simulink model "mcb_microchip_pmsm_foc_sensorless_dsPIC33EP256MC506"  (R2021b)
settings: Solver=FixedStepDiscrete  StartTime=0.0  StopTime=10  FixedStep=Ts  RelTol=1e-3  EnableMultiTasking=on
InitFcn:
  | mcb_microchip_pmsm_foc_sensorless_dsPIC33_data;
values from neighbouring files (symbols this model uses):
  dataType = fixdt(1,16,14)    [mcb_microchip_pmsm_foc_sensorless_dsPIC33_data.m]    (also in mcb_pmsm_foc_sensorless_dsPIC33_data.m)
  dataType2 = fixdt(1,16,12)    [mcb_microchip_pmsm_foc_sensorless_dsPIC33_data.m]    (also in mcb_pmsm_foc_sensorless_dsPIC33_data.m)
  PI_params = mcb.internal.SetControllerParameters(pmsm,inverter,PU_System,T_pwm,Ts,Ts_speed)    [mcb_microchip_pmsm_foc_sensorless_dsPIC33_data.m]    (also in mcb_pmsm_foc_sensorless_dsPIC33_data.m)
  PU_System = mcb_SetPUSystem(pmsm,inverter)    [mcb_microchip_pmsm_foc_sensorless_dsPIC33_data.m]    (also in mcb_pmsm_foc_sensorless_dsPIC33_data.m)
  PWM_frequency = 20e3    (= 20000)    [mcb_microchip_pmsm_foc_sensorless_dsPIC33_data.m]    (also in mcb_pmsm_foc_sensorless_dsPIC33_data.m)
  Speed_openLoop_PU = 0.1    [mcb_microchip_pmsm_foc_sensorless_dsPIC33_data.m]    (also in mcb_pmsm_foc_sensorless_dsPIC33_data.m)
  Ts = T_pwm    (= 5e-05)    [mcb_microchip_pmsm_foc_sensorless_dsPIC33_data.m]    (also in mcb_pmsm_foc_sensorless_dsPIC33_data.m)
  Ts_speed = 30*Ts    (= 0.0015)    [mcb_microchip_pmsm_foc_sensorless_dsPIC33_data.m]    (also in mcb_pmsm_foc_sensorless_dsPIC33_data.m)
undefined symbols (not defined in the file or in its folder): A4, C5, D8, F1, inverter, P20, P53, P97, Pin, pmsm, PWMmax
libraries: MCHP_Blockset x16, mcbcontrolslib x13, simulink x9, mcbpositiondecoderlib x2, mcbplantlib x1, autolibpmsmexterior x1
(part 2 of 3)

== system mcb_microchip_pmsm_foc_sensorless_dsPIC33EP256MC506/Current Control/PWM Driver ==
  PWM (abc) : Inport
  Dead time Compensation : Bias  Bias=round( (inverter.deadtime/Ts) *PWMmax )
  Demux : Demux  Outputs=3
  PWM High Speed : MCHP_Blockset/PWM IO/PWM High Speed  pop1=[1]  chk1="[1  1  1  0  0]"  chkHL1="[1  1  1  1  1  1  1  1 ; 1  1  1  1  1  1  1  1]"  maxP1={ 'Ts','5e-05','5e-05','0.001','0.001','0.001','0.001','0.001';'0.001','0.001','1e-06','0.001','0.001','0.001','0.001','0.001'}  InitP2={ 'Ts','5e-05','5e-05','0.001','0.001','0.001','0.001','0.001';'0.001','0.001','0.001','0.001','0.001','0.001','0.001','0.001'}  chkP2="[0  0  0  1  1  1  1  1 ; 1  0  0  1  1  1  1  1]"  InitDC={ '4','4','4','50','50','50','50','50';'0.001','0.001','0.001','50','50','50','50','50'}  chkDC="[1  1  1  1  1  1  1  1 ; 0  0  0  1  1  1  1  1]"  InitPh={ '0','0','0','0.001','0.001','0.001','0.001','0.001';'0','0','0','0.001','0.001','0.001','0.001','0.001'}  chkPh="[0  0  0  1  1  1  1  1 ; 0  0  0  1  1  1  1  1]"  edSEvTrigx={ '0','-1','-1','-1','-1','-1','-1','-1'}  chkSEvTrigx="[0  0  0  1  1  1  1  1]"  popFlt="[2  2  2  1  1  1  1  1]"  popFltPin="[20  20  20   4   4   4   4   4]"  popFltPinRp="[1  1  1  1  1  1  1]"  popFltActivH="[2  2  2  1  1  1  1  1]"  popFltForceH="[2  2  2  2  2  2  2  2]"  popFltForceL="[1  1  1  1  1  1  1  1]"  chkFltBlkOut="[0  0  0  0  0  0  0  0]"  popIndepFaultMode="[1  1  1  1  1  1  1  1]"  popCurEnabled="[1  1  1  1  1  1  1  1]"  popCurPin="[4  31   4   4   4   4   4   4]"  popCurActiveH="[1  1  1  1  1  1  1  1]"  popCurForceH="[2  1  2  1  1  1  1  1]"  popCurForceL="[2  1  2  1  1  1  1  1]"  ChkCurBlkOut="[1  0  0  0  0  0  0  0]"  ChkCurBlkOutTime="[1  0  1  0  0  0  0  0]"  popBLANKSEL="[1  1  1  1  1  1  1  1]"  popBPHHBPHL="[1  1  1  1  1  1  1  1]"  popBPLHBPLL="[1  1  1  1  1  1  1  1]"  popFLTLEBEN_CLLEBEN="[1  1  1  1  1  1  1  1]"  popPHR_PHF="[2  1  1  1  1  1  1  1]"  popPLR_PLF="[3  1  1  1  1  1  1  1]"  edLEB={ '100e-9','50e-9','150e-9','50e-9','50e-9','50e-9','50e-9','50e-9'}  popDT="[1  1  1  3  3  3  3  3]"  edDTRx={ '0','0','0','1e-05','1e-05','1e-05','1e-05','1e-05'}  edAltDTRx={ 'inverter.deadtime','inverter.deadtime','inverter.deadtime','1e-05','1e-05','1e-05','1e-05','1e-05'}  S_INPUT="[5  5  5]"  S_INPUT_Size="[1  1  1]"  S_OUTPUT=[]  S_OUTPUT_Size=[]  S_DWORK_Type=[]  S_DWORK_Size=[]  ADC_VARTRIG={PWM Primary Special Event Trigger;6}  evalin_ws=PWMmax = 3499;PWM1max = 3499;PWM2max = 3499;PWM3max = 3499;  SampleTime=-1  ORDERING=None  MCHP_PORT={PWM1 Fault}{FLT32}4:0:B4;{PWM2 Fault}{FLT32}4:0:B4;{PWM3 Fault}{FLT32}4:0:B4;{PWM1H}{PWM1H}4:4:B14;{PWM1L}{PWM1L}4:4:B15;{PWM2H}{PWM2H}4:4:B12;{PWM2L}{PWM2L}4:4:B13;{PWM3H}{PWM3H}4:4:B10;{PWM3L}{PWM3L}4:4:B11;  MCHP_MASTERLINK=mcb_pmsm_foc_sensorless_dsPIC33EP256MC506/Hardware Init/Microchip Master  MCHP_VERSION=v3.38  Parameter50=0
      settings: SourceProductName=MPLAB Device Blocks for Simulink
  Saturation low side turn on errate workaround + errata for Phase shift (times 2) : Saturate  UpperLimit=PWMmax  LowerLimit=round( (inverter.deadtime/Ts) *PWMmax )* 2
  int to uint : DataTypeConversion  OutDataTypeStr=uint16  ConvertRealWorld=Stored Integer (SI)
  wires:
  int to uint/1 -> Saturation low side turn on errate workaround + errata for Phase shift (times 2)/1
  Dead time Compensation/1 -> int to uint/1
  PWM (abc)/1 -> Dead time Compensation/1
  Saturation low side turn on errate workaround + errata for Phase shift (times 2)/1 -> Demux/1
  Demux/1 -> PWM High Speed/1
  Demux/2 -> PWM High Speed/2
  Demux/3 -> PWM High Speed/3

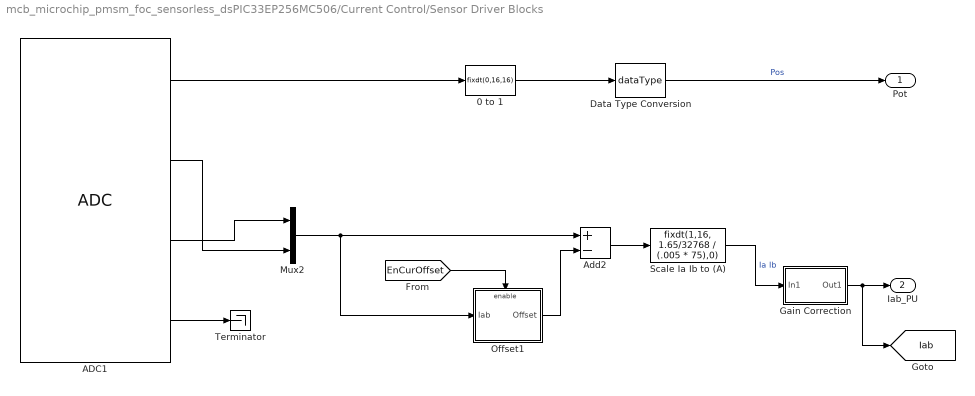
== system mcb_microchip_pmsm_foc_sensorless_dsPIC33EP256MC506/Current Control/Sensor Driver Blocks ==
  0 to 1 : DataTypeConversion  OutDataTypeStr=fixdt(0,16,16)  ConvertRealWorld=Stored Integer (SI)
  ADC1 : MCHP_Blockset/Analog IO/ADC  Priority=5  ADC_REF=1  Mode=10 bits (allows exact simultaneous sampling)  FORM=dddd dddd dddd 0000 ==> Unsigned fractional  ADC_R="< 5    kOhm"  nSAMPLECHANNELS=CH0 : CH1 : CH2 : CH3  nSAMPLECHANNELS_12bits=CH0 only  SIMULTANEOUS=Simultaneously on all Channels  ADxCSS=[13]  MUXA_CH0N=off  MUXA_CH123=Dynamic Options  MUXA_CH123_TXT=AN0 : AN1 : AN2  MUXB_CH0=AN13  MUXB_CH0N=on  MUXB_CH123=Dynamic Options  MUXB_CH123_TXT=AN0 : AN1 : AN2  SequenceRepeat=1  SequenceTiming=are done as fast as possible ; triggered by user define source  SSRC_SSRCG=Dynamic Options  SSRC_SSRCG_TXT=6  Update_BlockOutput=After each trig and conversion sequence  Trig_TimeStep=with each update of the ADC block output  ADC_DMA_CHANNEL=Use Interrupt instead of DMA  SampleTime=5e-05  Info=Total Time for Sample & Conversion : 4.4571e-06s including 3.4286e-07s (x 1) sample time.  MCHP_PORT={Analog Input 0}{AN0}15:2:A0;{Analog Input 1}{AN1}15:2:A1;{Analog Input 2}{AN2}15:2:B0;{Analog Input 13}{AN13}15:2:E13;  MCHP_MASTERLINK=mcb_pmsm_foc_sensorless_dsPIC33EP256MC506/Hardware Init/Microchip Master  ADC_TIMING=[4.4571428571428571832e-06]
      settings: SourceProductName=MPLAB Device Blocks for Simulink
  Add2 : Sum  Inputs=+-  OutDataTypeStr=int16  RndMeth=Zero
  Data Type Conversion : DataTypeConversion  OutDataTypeStr=dataType  RndMeth=Simplest
  Gain Correction : Subsystem
  Mux2 : Mux  Inputs=2
  Offset1 : Subsystem
  Scale Ia Ib to (A) : DataTypeConversion  OutDataTypeStr=fixdt(1,16, 1.65/32768 / (.005 * 75),0)  ConvertRealWorld=Stored Integer (SI)  RndMeth=Zero
  Terminator : Terminator
  Pot : Outport  VectorParamsAs1DForOutWhenUnconnected=off
  Iab_PU : Outport  Port=2  VectorParamsAs1DForOutWhenUnconnected=off
  tag scope: Iab=global
  wires:
  Mux2/1 -> Offset1/1(Iab), Add2/1
  0 to 1/1 -> Data Type Conversion/1
  [EnCurOffset] -> Offset1/Enable
  Data Type Conversion/1 -> Pot/1  "Pos"
  Add2/1 -> Scale Ia Ib to (A)/1
  ADC1/3 -> Mux2/1
  ADC1/1 -> 0 to 1/1
  Offset1/1(Offset) -> Add2/2
  ADC1/2 -> Mux2/2
  ADC1/4 -> Terminator/1
  Scale Ia Ib to (A)/1 -> Gain Correction/1(In1)  "Ia Ib"
  Gain Correction/1(Out1) -> [Iab], Iab_PU/1

== system mcb_microchip_pmsm_foc_sensorless_dsPIC33EP256MC506/Current Control/To Matlab Host  ==
  note: Note: Uncomment above blocks and comment Serial Send (below) to use Microchip's picgui interface to log hardware signals
  speed : Inport
  Data Store Read2 : DataStoreRead  DataStoreName=Speed_ref  IndexOptions=Index vector (dialog)  Indices=1  OutputSizes=1
  Gain : Gain  Gain=PU_System.N_base  OutDataTypeStr=uint16  RndMeth=Simplest
  Gain1 : Gain  Gain=PU_System.N_base  OutDataTypeStr=uint16
  Serial Send : Subsystem
  UART Tx-Matlab : MCHP_Blockset/BUS UART/UART Tx-Matlab  Commented=on  UART_REF=2  CHANNELS=[1 2]  AllOrNothing=off  SampleTime=.001  MCHP_MASTERLINK=mcb_pmsm_foc_sensorless_dsPIC33EP256MC506/Hardware Init/Microchip Master  MCHP_COMPILED_INFO="CompiledSampleTime= [0.0010000000000000000208   0 ];CompiledInportDataTypes=[  4   4 ];CompiledInportDataWidth=[1  1];"
      settings: SourceProductName=MPLAB Device Blocks for Simulink
  int to uint2 : DataTypeConversion  OutDataTypeStr=int16  ConvertRealWorld=Stored Integer (SI)
  int to uint3 : DataTypeConversion  OutDataTypeStr=int16  ConvertRealWorld=Stored Integer (SI)
  picgui Graphical interface : MCHP_Blockset/BUS UART/picgui Graphical interface  Commented=on  Nothing=0
      settings: SourceProductName=MPLAB Device Blocks for Simulink
  wires:
  speed/1 -> Serial Send/2(Speed_fb), Gain1/1
  Data Store Read2/1 -> Serial Send/1(Speed_ref), Gain/1
  Gain/1 -> int to uint3/1
  Gain1/1 -> int to uint2/1
  int to uint3/1 -> UART Tx-Matlab/1  "U2 CH1"
  int to uint2/1 -> UART Tx-Matlab/2  "U2 CH2"

== system mcb_microchip_pmsm_foc_sensorless_dsPIC33EP256MC506/Hardware Init/Open Board and Motor pages ==

== system mcb_microchip_pmsm_foc_sensorless_dsPIC33EP256MC506/Inverter and Motor/Codegeneration ==
  Duty_Cycles : Inport
  Ground : Ground
  Terminator : Terminator
  Feedbacks_Iab : Outport  VectorParamsAs1DForOutWhenUnconnected=off
  wires:
  Ground/1 -> Feedbacks_Iab/1
  Duty_Cycles/1 -> Terminator/1

== system mcb_microchip_pmsm_foc_sensorless_dsPIC33EP256MC506/Inverter and Motor/Simulation ==
  Duty_Cycles : Inport
  Inverter : Subsystem
  Load_Profile (Torque) : Subsystem
  Sensor_Measurements : Subsystem
  Surface Mount PMSM : autolibpmsmexterior/Surface Mount PMSM  port_config=Torque  sim_type=Discrete  Ts=Ts  P=pmsm.p  Rs=pmsm.Rs + inverter.R_board  Ldq_=pmsm.Ld  KConstText=Permanent flux linkage constant (lambda_pm):  lambda_pm=pmsm.FluxPM  Ke=159.9771  Kt=1.323  mechanical=[pmsm.J, pmsm.B, 0]  idq0=[0 0]  theta_init=0  omega_init=0  KConst=pmsm.FluxPM  lambda_pm_calc=pmsm.FluxPM  RefBlkName='autolibpmsmexterior/Surface Mount PMSM'  aMode=5  Ldq="[0.0002      0.0002]"
      settings: SourceProductBaseCode=PW,DR,MT,UV,VE
  Terminator : Terminator
  Terminator1 : Terminator
  Feedbacks_Iab : Outport  VectorParamsAs1DForOutWhenUnconnected=off
  wires:
  Surface Mount PMSM/3 -> Terminator/1
  Duty_Cycles/1 -> Inverter/1(Duty_abc)
  Surface Mount PMSM/2 -> Sensor_Measurements/1(PhaseCurr)  "Iabc"
  Sensor_Measurements/1(Iab_fb) -> Feedbacks_Iab/1
  Load_Profile (Torque)/1(Load_Trq) -> Surface Mount PMSM/1
  Inverter/1(Vabc) -> Surface Mount PMSM/2
  Surface Mount PMSM/1 -> Terminator1/1

== system mcb_microchip_pmsm_foc_sensorless_dsPIC33EP256MC506/Speed Control/PI_Controller_Speed ==
  N_ref : Inport
  N_fb : Inport  Port=2
  Enable : EnablePort
  AND : Logic  IconShape=distinctive  AllPortsSameDT=off  OutDataTypeStr=boolean
  Data Store Read : DataStoreRead  DataStoreName=Enable  IndexOptions=Index vector (dialog)  Indices=1  OutputSizes=1
  Data Store Read1 : DataStoreRead  DataStoreName=EnableFOC  IndexOptions=Index vector (dialog)  Indices=1  OutputSizes=1
  Discrete PI Controller with anti-windup & reset : mcbcontrolslib/Discrete PI Controller  with anti-windup & reset  UpperSaturationLimit=1  LowerSaturationLimit=-1
      settings: SourceProductBaseCode=MT
  Ki1 : Constant  Value=Ts_speed * PI_params.Ki_speed  OutDataTypeStr=dataType  SampleTime=-1
  Ki2 : Constant  Value=0  OutDataTypeStr=dataType  SampleTime=-1
  Kp1 : Constant  Value=PI_params.Kp_speed  OutDataTypeStr=dataType2  SampleTime=-1
  Logical Operator : Logic  Operator=NOT  IconShape=distinctive  AllPortsSameDT=off  OutDataTypeStr=boolean
  Sum : Sum  Inputs=|+-  OutDataTypeStr=Inherit: Same as first input
  Iq_ref : Outport  OutputWhenDisabled=reset  InitialOutput=0  VectorParamsAs1DForOutWhenUnconnected=off
  wires:
  Discrete PI Controller with anti-windup & reset/1 -> Iq_ref/1
  Ki1/1 -> Discrete PI Controller with anti-windup & reset/3
  Kp1/1 -> Discrete PI Controller with anti-windup & reset/2
  N_fb/1 -> Sum/2
  Sum/1 -> Discrete PI Controller with anti-windup & reset/1
  Logical Operator/1 -> Discrete PI Controller with anti-windup & reset/4
  Ki2/1 -> Discrete PI Controller with anti-windup & reset/5
  N_ref/1 -> Sum/1  "Speed_Ref"
  Data Store Read1/1 -> AND/1
  Data Store Read/1 -> AND/2
  AND/1 -> Logical Operator/1

== system mcb_microchip_pmsm_foc_sensorless_dsPIC33EP256MC506/Speed Control/Speed_Ref_Selector ==
  Speed_Ref : Inport
  Constant : Constant  Value=Speed_openLoop_PU  OutDataTypeStr=dataType
  Data Store Read1 : DataStoreRead  DataStoreName=EnClosedLoop  IndexOptions=Index vector (dialog)  Indices=1  OutputSizes=1
  Switch : Switch  Criteria=u2 > Threshold
  Zero_Cancellation : mcbcontrolslib/IIR Filter  VariantControl=Low Pass Filter  VariantSelect=Low-pass  Filter_constant=0.2  advancedSettings=off  Ts=50e-6  cutOff_freq=795.7747
      settings: SourceProductBaseCode=MT
  Speed_ref : Outport
  wires:
  Constant/1 -> Switch/3
  Data Store Read1/1 -> Switch/2
  Switch/1 -> Zero_Cancellation/1
  Speed_Ref/1 -> Switch/1
  Zero_Cancellation/1 -> Speed_ref/1

== system mcb_microchip_pmsm_foc_sensorless_dsPIC33EP256MC506/System Inputs/Adjust Pot output ==
  note: Toggle between enable and disable on press on Button S2
  In1 : Inport
  Add : Sum
  Button S2 : MCHP_Blockset/Digital IO/Digital Input  PORT=Dynamic Options  PORT_TXT="G   [ 6 : 9 ]"  PIN=7  PACK=off  SIMULTANEOUS=off  ORDERING=None  SampleTime=-1  MCHP_PORT={Digital In}{DIN}2:0:G7;  MCHP_MASTERLINK=mcb_pmsm_foc_sensorless_dsPIC33EP256MC506/Hardware Init/Microchip Master
      settings: SourceProductName=MPLAB Device Blocks for Simulink
  Constant : Constant  Value=0.3
  Gain : Gain  Gain=0.45
  Saturation : Saturate  UpperLimit=0.75  LowerLimit=0.3
  Triggered Subsystem : Subsystem  TreatAsAtomicUnit=on
  Out1 : Outport
  wires:
  In1/1 -> Gain/1
  Constant/1 -> Add/2
  Gain/1 -> Add/1
  Add/1 -> Saturation/1
  Saturation/1 -> Out1/1
  Button S2/1 -> Triggered Subsystem/Trigger

== system mcb_microchip_pmsm_foc_sensorless_dsPIC33EP256MC506/System Inputs/Sim ==
  Data Store Write : DataStoreWrite  DataStoreName=Enable  IndexOptions=Index vector (dialog)  Indices=1  OutputSizes=1
  Data Type Conversion : DataTypeConversion
  Enable : Step  Time=0.5  SampleTime=0
  Speed Ref (Sim) : Step  Time=4  Before=0.5  After=0.75  OutDataTypeStr=Inherit: Inherit via back propagation
  Out1 : Outport
  wires:
  Speed Ref (Sim)/1 -> Out1/1
  Data Type Conversion/1 -> Data Store Write/1
  Enable/1 -> Data Type Conversion/1

== system mcb_microchip_pmsm_foc_sensorless_dsPIC33EP256MC506/Current Control/Closed Loop Control/Clarke Transform ==
  a : Inport
  b : Inport  Port=2
  Data Type Duplicate : DataTypeDuplicate
  a16 : AlgorithmDescriptor  AlgorithmName=mcb_clarke  NumberOfInputs=2  InputBlockPath1=a  InputBlockPath2=b  InputBlockPath3=sine  InputBlockPath4=cos  ParameterBlockPath1=Constant  ParameterName1=Value  NumberOfOutputs=2  OutputBlockPath1=Alpha  OutputBlockPath2=Beta  AlgorithmParameterName1=AxisAlignment  AlgorithmParameterValue1=dAxis  AlgorithmParameterPrimary1=on
  a_plus_2b : Sum  Inputs=+++  RndMeth=Zero  OutDataTypeStr=Inherit: Same as first input
  one_by_sqrt3 : Gain  Gain=1/sqrt(3)  RndMeth=Zero  OutDataTypeStr=Inherit: Same as input
  Alpha : Outport  VectorParamsAs1DForOutWhenUnconnected=off
  Beta : Outport  Port=2  VectorParamsAs1DForOutWhenUnconnected=off
  wires:
  a/1 -> a_plus_2b/1, Alpha/1, Data Type Duplicate/1
  one_by_sqrt3/1 -> Beta/1
  a_plus_2b/1 -> one_by_sqrt3/1
  b/1 -> a_plus_2b/2, a_plus_2b/3, Data Type Duplicate/2

== system mcb_microchip_pmsm_foc_sensorless_dsPIC33EP256MC506/Current Control/Closed Loop Control/Current_Controllers ==
  Id : Inport
  Iq : Inport  Port=2
  Idq_ref_PU : Inport  Port=3
  DQ Limiter : mcbcontrolslib/DQ Limiter  Vmax=0.95
      settings: SourceProductBaseCode=MT
  Demux : Demux  Outputs=2
  Mux : Mux
  PI_Controller_Id : Subsystem
  PI_Controller_Iq : Subsystem
  Terminator : Terminator
  Vd_ref : Outport  VectorParamsAs1DForOutWhenUnconnected=off
  Vq_ref : Outport  Port=2  VectorParamsAs1DForOutWhenUnconnected=off
  Idq : Outport  Port=3  VectorParamsAs1DForOutWhenUnconnected=off
  wires:
  Iq/1 -> Mux/4, PI_Controller_Iq/2(I_fb)  "Iq_fb"
  Id/1 -> Mux/2, PI_Controller_Id/2(I_fb)  "Id_fb"
  Demux/1 -> Mux/1, PI_Controller_Id/1(I_ref)  "Id_Ref"
  Demux/2 -> Mux/3, PI_Controller_Iq/1(I_ref)  "Iq_Ref"
  Idq_ref_PU/1 -> Demux/1
  DQ Limiter/3 -> Terminator/1
  Mux/1 -> Idq/1
  PI_Controller_Iq/1(V_ref) -> DQ Limiter/2
  PI_Controller_Id/1(V_ref) -> DQ Limiter/1
  DQ Limiter/1 -> Vd_ref/1
  DQ Limiter/2 -> Vq_ref/1

== system mcb_microchip_pmsm_foc_sensorless_dsPIC33EP256MC506/Current Control/Closed Loop Control/Open_Loop_Control ==
  Pos_PU : Inport
  Speed_fb : Inport  Port=2
  Constant : Constant  Value=Speed_openLoop_PU  OutDataTypeStr=dataType
  Gain : Gain  Gain=Ts*PU_System.N_base*pmsm.p/60  OutDataTypeStr=Inherit: Same as input  ParamDataTypeStr=Inherit: Same as input
  OpentoClosed : Subsystem
  Position Generator : mcbcontrolslib/Position Generator  AngleOutput=Per-unit  ThetaSource=External  ThetaInput=5e-4  DataType=double  ExternalReset=none  Offset=0
      settings: SourceProductBaseCode=MT
  Switch : Switch  Criteria=u2 ~= 0
  Pos_PU_Out : Outport
  wires:
  Position Generator/1 -> Switch/3  "Eps"
  Gain/1 -> Position Generator/1
  Switch/1 -> Pos_PU_Out/1
  Pos_PU/1 -> Switch/1
  Constant/1 -> Gain/1
  Speed_fb/1 -> OpentoClosed/1(Speed_fb)
  OpentoClosed/1(EnClosedLoop) -> Switch/2

== system mcb_microchip_pmsm_foc_sensorless_dsPIC33EP256MC506/Current Control/Input Scaling/DC component removal ==
  SigIN : Inport
  Data Type Conversion1 : DataTypeConversion  OutDataTypeStr=dataType  RndMeth=Zero
  High Pass Filter 1 : Subsystem  Tag=FilterWizardSubSystem
  SigOUT : Outport
  wires:
  SigIN/1 -> High Pass Filter 1/1(Input)
  High Pass Filter 1/1(Output) -> Data Type Conversion1/1
  Data Type Conversion1/1 -> SigOUT/1

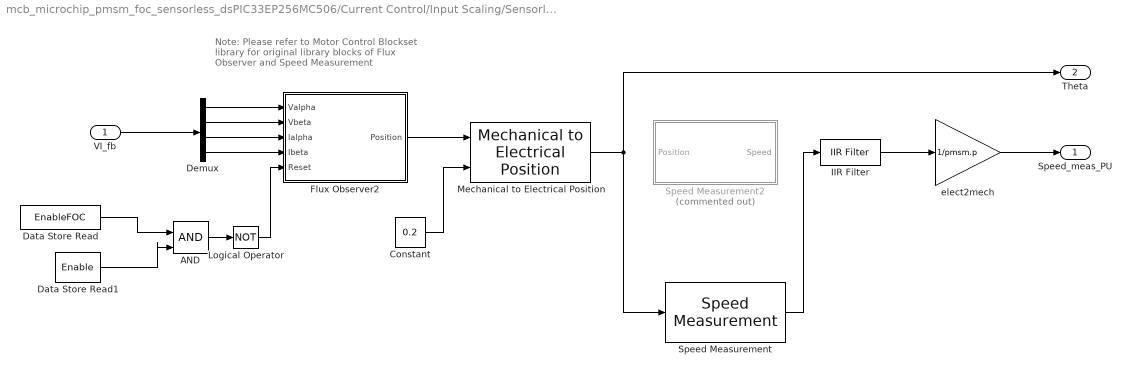
== system mcb_microchip_pmsm_foc_sensorless_dsPIC33EP256MC506/Current Control/Input Scaling/Sensorless ==
  note: Note: Please refer to Motor Control Blockset library for original library blocks of Flux Observer and Speed Measurement
  VI_fb : Inport
  AND : Logic  IconShape=distinctive  AllPortsSameDT=off  OutDataTypeStr=boolean
  Constant : Constant  Value=0.2  OutDataTypeStr=dataType
  Data Store Read : DataStoreRead  DataStoreName=EnableFOC  IndexOptions=Index vector (dialog)  Indices=1  OutputSizes=1
  Data Store Read1 : DataStoreRead  DataStoreName=Enable  IndexOptions=Index vector (dialog)  Indices=1  OutputSizes=1
  Demux : Demux
  Flux Observer2 : Subsystem  AncestorBlock=mcbpositiondecoderlib/Flux Observer  mask(Flux Observer){MotorSelection=PMSM, BlockInputUnit=Per-unit, PerUnitVoltage=PU_System.V_base, PerUnitCurrent=PU_System.I_base, PositionSelect=on, FluxSelect=off, TorqueSelect=off, PolePairs=4, StatorResistance=pmsm.Rs, StatorDAxisInductance=pmsm.Ld, StatorLeakageInductance=0.0068, RotorLeakageInductance=0.0068, MagnetizingInductance=0.0300, CutoffFreq=3.1863, BlockSampleTime=Ts, PositionUnit=Per-unit, PositionDatatype=dataType, FluxUnit=Weber, PerUnitFlux=0.1, FluxDatatype=single, TorqueUnit=Nm, PerUnitTorque=100, TorqueDatatype=single}
      mask prompts: MotorSelection "Motor selection:"; BlockInputUnit "Input units:"; PerUnitVoltage "Base voltage (V):"; PerUnitCurrent "Base current (A):"; PositionSelect "Position"; FluxSelect "Flux"; TorqueSelect "Torque"; PolePairs "Pole pairs:"; StatorResistance "Stator resistance (ohm):"; StatorDAxisInductance "Stator d-axis inductance (H):"; StatorLeakageInductance "Stator leakage inductance (H):"; RotorLeakageInductance "Rotor leakage inductance (H):"; MagnetizingInductance "Magnetizing inductance (H):"; CutoffFreq "Cutoff frequency (Hz):"; BlockSampleTime "Discrete step size (s):"; PositionUnit "Position unit:"; PositionDatatype "Position datatype:"; FluxUnit "Flux unit:"; PerUnitFlux "Per unit flux (Wb):"; FluxDatatype "Flux datatype:"; TorqueUnit "Torque unit:"; PerUnitTorque "Per unit torque (Nm):"; TorqueDatatype "Torque datatype:"
      mask help:
      | <p>Compute &#952;<sub>e</sub> (electrical position), &#936; (rotor magnetic flux), and T<sub>e</sub> (electromechanical torque) of a Permanent Magnet Synchronous Machine (PMSM) or Alternating Current Induction Machine (ACIM) from the voltages and currents in the stationary reference frame.
      | <br><br>
      | Use the Input units parameter to select the input unit of the block.
      | <br><br>
      | Use the Cutoff frequency parameter to set the lower cutoff frequency of the internal high Pass filter. Ensure that the values for Base voltage and Base current conform to the maximum applicable limits for the FO.</p>
      mask init:
      | mcb.internal.FOCb('MaskInitFcn', gcbh);
      mask Help: eval('mcb.internal.helpview(''fluxobserver'')')
      mask TypeOptions MotorSelection: PMSM | ACIM
      mask Callback MotorSelection: mcb.internal.FOCb('MotorSelectionMaskDisplay', gcbh);
      mask TypeOptions BlockInputUnit: SI unit | Per-unit
      mask Callback BlockInputUnit: mcb.internal.FOCb('MaskDisplay', gcbh);
      mask Callback PositionSelect: mcb.internal.FOCb('MaskDisplay', gcbh);
      mask Callback FluxSelect: mcb.internal.FOCb('MaskDisplay', gcbh);
      mask Callback TorqueSelect: mcb.internal.FOCb('MaskDisplay', gcbh);
      mask TypeOptions PositionUnit: Radians | Degrees | Per-unit
      mask TypeOptions FluxUnit: Weber | Per-unit
      mask Callback FluxUnit: mcb.internal.FOCb('MaskDisplay', gcbh);
      mask TypeOptions TorqueUnit: Nm | Per-unit
      mask Callback TorqueUnit: mcb.internal.FOCb('MaskDisplay', gcbh);
      mask DialogControl Container4 Prompt: Motor Parameters
      mask DialogControl Container7 Prompt: Block Output
      mask DialogControl Container8 Prompt: Datatypes
      mask Display:
      | color('black');
      | port_label('input',1, 'V_{\alpha}', 'interpreter', 'tex');
      | port_label('input',2, 'V_{\beta}', 'interpreter', 'tex');
      | port_label('input',3, 'I_{\alpha}', 'interpreter', 'tex');
      | port_label('input',4, 'I_{\beta}', 'interpreter', 'tex');
      | port_label('input',5, 'Rst', 'interpreter', 'tex');
      | port_label('output',1, '\theta_{e}', 'interpreter', 'tex');
      | %No Flux;
      | %No Torque;
      | fprintf('Flux\nObserver');
  IIR Filter : mcbcontrolslib/IIR Filter  VariantControl=Low Pass Filter  VariantSelect=Low-pass  Filter_constant=0.02  advancedSettings=off  Ts=50e-6  cutOff_freq=64.9612
      settings: SourceProductBaseCode=MT
  Logical Operator : Logic  Operator=NOT  IconShape=distinctive  AllPortsSameDT=off  OutDataTypeStr=boolean
  Mechanical to Electrical Position : mcbpositiondecoderlib/Mechanical to Electrical Position  NrPP=1  selectedRange=Per unit  MechOfstInputType=Input port  mechOffsetIn=0  maxAngleIn=1  InputDataType=dataType  VariantSelect=floating-point
      settings: SourceProductBaseCode=MT
  Speed Measurement : mcbpositiondecoderlib/Speed Measurement  PositionUnit=Per unit  PositionScalingDatatype=uint16  SpeedCalculationMode=Time interval for speed calculation  SampleTimeAsync=Ts  MaximumApplicationSpeed=1000  SpeedResolution=5e-6  DelayLength=20  MaximumMeasurableSpeed=-0.98352  MeasurableSpeedResolution=5.0304e-07  SpeedUnit=Per unit based on dialog  PerUnitSpeed=PU_System.N_base  SpeedDataType=dataType2
      settings: SourceProductBaseCode=MT
  Speed Measurement2 : Subsystem  Commented=on  AncestorBlock=mcbpositiondecoderlib/Speed Measurement  mask(Speed Measurement){PositionUnit=Per unit, SpeedCalculationMode=Time interval for speed calculation, SampleTimeAsync=Ts, MaximumApplicationSpeed=1000, SpeedResolution=5e-6, DelayLength=20, MaximumMeasurableSpeed=29999, MeasurableSpeedResolution=1.397e-05, SpeedUnit=Per unit based on dialog, PerUnitSpeed=PU_System.N_base, SpeedDataType=dataType2}
      mask prompts: PositionUnit "Position unit:"; SpeedCalculationMode "Speed calculation criteria:"; SampleTimeAsync "Discrete step size (s):"; MaximumApplicationSpeed "Maximum application speed (RPM):"; SpeedResolution "Speed resolution (RPM):"; DelayLength "Delays for speed calculation (number of samples):"; MaximumMeasurableSpeed "Maximum measurable speed (RPM):"; MeasurableSpeedResolution "Measurable speed resolution (RPM):"; SpeedUnit "Speed unit:"; PerUnitSpeed "Per unit speed (RPM):"; SpeedDataType "Speed data type:"
      mask help:
      | <p>Compute the speed from the rotor angular position.
      | <br>
      | <br>
      | &#952; (position) port accepts the position signal as either scalar fixed point or scalar floating point data type.</P>
      mask init:
      | mcb.internal.SpeedMeasurementCb('SpeedToCount', gcbh);
      | mcb.internal.SpeedMeasurementCb('SpeedUnit', gcbh);
      | mcb.internal.SpeedMeasurementCb('SetMaskDisplay', gcbh);
      mask Help: eval('mcb.internal.helpview(''speedmeasurement'')')
      mask TypeOptions PositionUnit: Radians | Degrees | Per unit
      mask Callback PositionUnit: mcb.internal.SpeedMeasurementCb('SpeedToCount', gcbh);
      mask TypeOptions SpeedCalculationMode: Maximum application speed | Speed resolution | Time interval for speed calculation
      mask Callback SpeedCalculationMode:
      | mcb.internal.SpeedMeasurementCb('SpeedCalculationModeCb', gcbh);
      | mcb.internal.SpeedMeasurementCb('MaskCalculation', gcbh,'SpeedCalculationMode');
      mask Callback SampleTimeAsync: mcb.internal.SpeedMeasurementCb('MaskCalculation', gcbh, 'SampleTimeAsync');
      mask Callback MaximumApplicationSpeed: mcb.internal.SpeedMeasurementCb('MaskCalculation', gcbh, 'MaximumApplicationSpeed');
      mask Callback SpeedResolution: mcb.internal.SpeedMeasurementCb('MaskCalculation', gcbh, 'SpeedResolution');
      mask Callback DelayLength: mcb.internal.SpeedMeasurementCb('MaskCalculation', gcbh, 'DelayLength');
      mask TypeOptions SpeedUnit: Degrees/Sec | Radians/Sec | RPM | Per unit based on maximum measurable speed | Per unit based on dialog
      mask Callback SpeedUnit: mcb.internal.SpeedMeasurementCb('PerUnitSpeedVisibility', gcbh);
      mask DialogControl General Prompt: Parameters
      mask Display:
      | color('black');
      | port_label('input',1, '\theta', 'texmode', 'on' );
      | port_label('output',1, '\omega', 'texmode', 'on' );
      | fprintf('Speed\nMeasurement');
  elect2mech : Gain  Gain=1/pmsm.p  OutDataTypeStr=dataType  RndMeth=Simplest
  Speed_meas_PU : Outport
  Theta : Outport  Port=2
  wires:
  Demux/3 -> Flux Observer2/3(Ialpha)
  Demux/1 -> Flux Observer2/1(Valpha)
  VI_fb/1 -> Demux/1
  Demux/4 -> Flux Observer2/4(Ibeta)
  Demux/2 -> Flux Observer2/2(Vbeta)
  IIR Filter/1 -> elect2mech/1
  elect2mech/1 -> Speed_meas_PU/1
  Speed Measurement/1 -> IIR Filter/1
  AND/1 -> Logical Operator/1
  Data Store Read/1 -> AND/1
  Data Store Read1/1 -> AND/2
  Flux Observer2/1(Position) -> Mechanical to Electrical Position/1
  Logical Operator/1 -> Flux Observer2/5(Reset)
  Mechanical to Electrical Position/1 -> Speed Measurement/1, Theta/1
  Constant/1 -> Mechanical to Electrical Position/2

== system mcb_microchip_pmsm_foc_sensorless_dsPIC33EP256MC506/Current Control/Output Scaling/Mode Selector ==
  Delay : Delay  DelayLength=1
  NOT : Logic  Operator=NOT  IconShape=distinctive  AllPortsSameDT=off  OutDataTypeStr=boolean
  Subsystem1 : Subsystem
  Up Counter : Subsystem
  CurrentOffsetEn : Outport
  wires:
  Up Counter/1(Count) -> Subsystem1/1(Count)
  Delay/1 -> NOT/1
  NOT/1 -> Up Counter/Enable
  Subsystem1/2(EnClosedLoop) -> Delay/1
  Subsystem1/1(Current Offset) -> CurrentOffsetEn/1

== system mcb_microchip_pmsm_foc_sensorless_dsPIC33EP256MC506/Current Control/Sensor Driver Blocks/Gain Correction ==
  In1 : Inport
  Demux : Demux  Outputs=2
  Gain : Gain  Gain=0.9615  RndMeth=Zero  OutDataTypeStr=Inherit: Same as input
  Mux : Mux  Inputs=2
  To Per-Unit : Gain  Gain=inverter.invertingAmp/PU_System.I_base  OutMin=-1  OutMax=1  OutDataTypeStr=fixdt(1,16)  RndMeth=Zero
  Out1 : Outport
  wires:
  Demux/1 -> Gain/1
  Demux/2 -> Mux/2
  To Per-Unit/1 -> Demux/1
  Gain/1 -> Mux/1
  Mux/1 -> Out1/1
  In1/1 -> To Per-Unit/1

== system mcb_microchip_pmsm_foc_sensorless_dsPIC33EP256MC506/Current Control/Sensor Driver Blocks/Offset1 ==
  Iab : Inport
  Enable : EnablePort
  Offset : Outport
  wires:
  Iab/1 -> Offset/1

== system mcb_microchip_pmsm_foc_sensorless_dsPIC33EP256MC506/Current Control/To Matlab Host /Serial Send ==
  Speed_ref : Inport
  Speed_fb : Inport  Port=2
  Debug_Data : Subsystem
  SCI_Tx : Subsystem
  wires:
  Debug_Data/1(Data_log) -> SCI_Tx/1(Data_Log)
  Speed_fb/1 -> Debug_Data/2(In2)
  Speed_ref/1 -> Debug_Data/1(In1)

== system mcb_microchip_pmsm_foc_sensorless_dsPIC33EP256MC506/Inverter and Motor/Simulation/Inverter ==
  Duty_abc : Inport
  Average-Value Inverter : mcbplantlib/Average-Value Inverter
  Constant2 : Constant  Value=inverter.V_dc  OutDataTypeStr=single  SampleTime=-1
  Data Type Conversion1 : DataTypeConversion  OutDataTypeStr=single  RndMeth=Simplest
  Vabc : Outport  VectorParamsAs1DForOutWhenUnconnected=off
  wires:
  Average-Value Inverter/1 -> Vabc/1
  Data Type Conversion1/1 -> Average-Value Inverter/1
  Duty_abc/1 -> Data Type Conversion1/1
  Constant2/1 -> Average-Value Inverter/2

== system mcb_microchip_pmsm_foc_sensorless_dsPIC33EP256MC506/Inverter and Motor/Simulation/Load_Profile (Torque) ==
  Constant : Constant  Value=0.2 * pmsm.T_rated  OutDataTypeStr=Inherit: Inherit via back propagation
  Data Type Conversion : DataTypeConversion  OutDataTypeStr=single
  IIR Filter : mcbcontrolslib/IIR Filter  VariantControl=Low Pass Filter  VariantSelect=Low-pass  Filter_constant=0.0001  advancedSettings=off  Ts=50e-6  cutOff_freq=0.31834
      settings: SourceProductBaseCode=MT
  Load_Trq : Outport  VectorParamsAs1DForOutWhenUnconnected=off
  wires:
  IIR Filter/1 -> Load_Trq/1
  Data Type Conversion/1 -> IIR Filter/1
  Constant/1 -> Data Type Conversion/1

== system mcb_microchip_pmsm_foc_sensorless_dsPIC33EP256MC506/Inverter and Motor/Simulation/Sensor_Measurements ==
  note: Delays
  note: Scaling
  PhaseCurr : Inport
  Data Type Conversion4 : DataTypeConversion  OutDataTypeStr=single  RndMeth=Simplest
  Delay1 : Delay  DelayLength=PI_params.delay_Currents
  Inverting OpAmp : Gain  Gain=1/PU_System.I_base  OutDataTypeStr=dataType  RndMeth=Simplest
  Selector : Selector  InputPortWidth=3  IndexOptions=Index vector (dialog)  Indices=[1 2]  OutputSizes=1
  Iab_fb : Outport  VectorParamsAs1DForOutWhenUnconnected=off
  wires:
  Selector/1 -> Inverting OpAmp/1
  PhaseCurr/1 -> Data Type Conversion4/1
  Data Type Conversion4/1 -> Delay1/1
  Delay1/1 -> Selector/1  "Iab_fb"
  Inverting OpAmp/1 -> Iab_fb/1

== system mcb_microchip_pmsm_foc_sensorless_dsPIC33EP256MC506/System Inputs/Adjust Pot output/Triggered Subsystem ==
  Trigger : TriggerPort  TriggerType=falling  VariantControl=Variant
  Data Store Write : DataStoreWrite  DataStoreName=Enable  IndexOptions=Index vector (dialog)  Indices=1  OutputSizes=1
  Delay : Delay  DelayLength=1  InitialCondition=0
  NOT : Logic  Operator=NOT  IconShape=distinctive  AllPortsSameDT=off  OutDataTypeStr=boolean
  wires:
  NOT/1 -> Data Store Write/1, Delay/1
  Delay/1 -> NOT/1

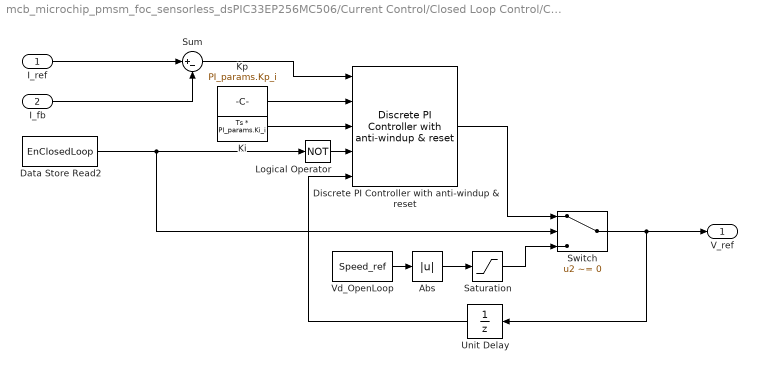
== system mcb_microchip_pmsm_foc_sensorless_dsPIC33EP256MC506/Current Control/Closed Loop Control/Current_Controllers/PI_Controller_Id ==
  I_ref : Inport
  I_fb : Inport  Port=2
  Abs : Abs  RndMeth=Simplest
  Data Store Read2 : DataStoreRead  DataStoreName=EnClosedLoop  IndexOptions=Index vector (dialog)  Indices=1  OutputSizes=1
  Discrete PI Controller with anti-windup & reset : mcbcontrolslib/Discrete PI Controller  with anti-windup & reset  UpperSaturationLimit=1  LowerSaturationLimit=-1
      settings: SourceProductBaseCode=MT
  Ki : Constant  Value=Ts * PI_params.Ki_i  OutDataTypeStr=dataType  SampleTime=-1
  Kp : Constant  Value=PI_params.Kp_i  OutDataTypeStr=dataType2  SampleTime=-1
  Logical Operator : Logic  Operator=NOT  IconShape=distinctive  AllPortsSameDT=off  OutDataTypeStr=boolean
  Saturation : Saturate  UpperLimit=0.15  LowerLimit=0.15  RndMeth=Simplest
  Sum : Sum  Inputs=|+-  OutDataTypeStr=Inherit: Same as first input
  Switch : Switch  Criteria=u2 ~= 0  RndMeth=Simplest
  Unit Delay : UnitDelay  SampleTime=-1  HasFrameUpgradeWarning=on
  Vd_OpenLoop : DataStoreRead  DataStoreName=Speed_ref  IndexOptions=Index vector (dialog)  Indices=1  OutputSizes=1
  V_ref : Outport  VectorParamsAs1DForOutWhenUnconnected=off
  wires:
  I_ref/1 -> Sum/1
  I_fb/1 -> Sum/2
  Data Store Read2/1 -> Switch/2, Logical Operator/1
  Sum/1 -> Discrete PI Controller with anti-windup & reset/1
  Kp/1 -> Discrete PI Controller with anti-windup & reset/2
  Ki/1 -> Discrete PI Controller with anti-windup & reset/3
  Logical Operator/1 -> Discrete PI Controller with anti-windup & reset/4
  Saturation/1 -> Switch/3
  Switch/1 -> Unit Delay/1, V_ref/1
  Discrete PI Controller with anti-windup & reset/1 -> Switch/1
  Unit Delay/1 -> Discrete PI Controller with anti-windup & reset/5
  Vd_OpenLoop/1 -> Abs/1
  Abs/1 -> Saturation/1

== system mcb_microchip_pmsm_foc_sensorless_dsPIC33EP256MC506/Current Control/Closed Loop Control/Current_Controllers/PI_Controller_Iq ==
  I_ref : Inport
  I_fb : Inport  Port=2
  Data Store Read1 : DataStoreRead  DataStoreName=EnClosedLoop  IndexOptions=Index vector (dialog)  Indices=1  OutputSizes=1
  Discrete PI Controller with anti-windup & reset : mcbcontrolslib/Discrete PI Controller  with anti-windup & reset  UpperSaturationLimit=1  LowerSaturationLimit=-1
      settings: SourceProductBaseCode=MT
  Ki : Constant  Value=Ts * PI_params.Ki_i  OutDataTypeStr=dataType  SampleTime=-1
  Kp : Constant  Value=PI_params.Kp_i  OutDataTypeStr=dataType2  SampleTime=-1
  Logical Operator : Logic  Operator=NOT  IconShape=distinctive  AllPortsSameDT=off  OutDataTypeStr=boolean
  Sum : Sum  Inputs=|+-  OutDataTypeStr=Inherit: Same as first input
  Switch : Switch  Criteria=u2 ~= 0  RndMeth=Simplest
  Unit Delay : UnitDelay  SampleTime=-1  HasFrameUpgradeWarning=on
  Vq_OpenLoop : Constant  Value=0  OutDataTypeStr=dataType  SampleTime=-1
  V_ref : Outport  VectorParamsAs1DForOutWhenUnconnected=off
  wires:
  I_fb/1 -> Sum/2
  I_ref/1 -> Sum/1
  Kp/1 -> Discrete PI Controller with anti-windup & reset/2
  Sum/1 -> Discrete PI Controller with anti-windup & reset/1
  Ki/1 -> Discrete PI Controller with anti-windup & reset/3
  Logical Operator/1 -> Discrete PI Controller with anti-windup & reset/4
  Data Store Read1/1 -> Switch/2, Logical Operator/1
  Vq_OpenLoop/1 -> Switch/3
  Discrete PI Controller with anti-windup & reset/1 -> Switch/1
  Unit Delay/1 -> Discrete PI Controller with anti-windup & reset/5
  Switch/1 -> Unit Delay/1, V_ref/1

== system mcb_microchip_pmsm_foc_sensorless_dsPIC33EP256MC506/Current Control/Closed Loop Control/Open_Loop_Control/OpentoClosed ==
  Speed_fb : Inport
  Chart : Stateflow chart  TreatAsAtomicUnit=on
  Data Store Read5 : DataStoreRead  DataStoreName=Enable  IndexOptions=Index vector (dialog)  Indices=1  OutputSizes=1
  Data Store Write1 : DataStoreWrite  DataStoreName=EnSpeedCtrl  IndexOptions=Index vector (dialog)  Indices=1  OutputSizes=1
  Data Store Write2 : DataStoreWrite  DataStoreName=EnClosedLoop  IndexOptions=Index vector (dialog)  Indices=1  OutputSizes=1
  Data Type Conversion : DataTypeConversion  OutDataTypeStr=boolean  RndMeth=Simplest
  Data Type Conversion1 : DataTypeConversion
  Enable Closed Loop : Constant  OutDataTypeStr=uint16
  Enable Closed Loop1 : Constant  Value=Speed_openLoop_PU*0.8  OutDataTypeStr=dataType
  Open Loop Start-up : Constant  Value=0  OutDataTypeStr=uint16
  Switch2 : Switch  Criteria=u2 > Threshold  Threshold=1
  EnClosedLoop : Outport
  wires:
  Open Loop Start-up/1 -> Switch2/3
  Data Store Read5/1 -> Chart/3(En)
  Chart/1(Mode) -> Switch2/2
  Switch2/1 -> Data Type Conversion/1
  Speed_fb/1 -> Chart/2(SpeedFb)
  Enable Closed Loop/1 -> Switch2/1
  Enable Closed Loop1/1 -> Chart/1(Limit)
  Data Type Conversion/1 -> EnClosedLoop/1, Data Store Write2/1
  Chart/2(SpeedCtrl) -> Data Type Conversion1/1
  Data Type Conversion1/1 -> Data Store Write1/1

== system mcb_microchip_pmsm_foc_sensorless_dsPIC33EP256MC506/Current Control/Input Scaling/DC component removal/High Pass Filter 1 ==
  Input : Inport
  A2Delay1 : Delay  DelayLength=1  InitialCondition=0
  B2Delay1 : Delay  DelayLength=1  InitialCondition=0
  CastStates1 : DataTypeConversion  OutDataTypeStr=fixdt(1,16,15)  SaturateOnIntegerOverflow=on  RndMeth=Zero
  ConvertIn : DataTypeConversion  OutDataTypeStr=fixdt(1,16,15)  RndMeth=Nearest  SaturateOnIntegerOverflow=on
  ConvertScale1 : DataTypeConversion  OutDataTypeStr=fixdt(1,16,15)  SaturateOnIntegerOverflow=on  RndMeth=Zero
  SumA21 : Sum  Inputs=|+-  AccumDataTypeStr=fixdt(1,32,27)  OutDataTypeStr=fixdt(1,32,27)  RndMeth=Zero  SaturateOnIntegerOverflow=on
  SumB21 : Sum  Inputs=|++  AccumDataTypeStr=fixdt(1,32,28)  OutDataTypeStr=fixdt(1,32,28)  RndMeth=Zero  SaturateOnIntegerOverflow=on
  a(2)(1) : Gain  Gain=-0.993965307066752457  ParamDataTypeStr=fixdt(1,16,14)  OutDataTypeStr=fixdt(1,32,29)  RndMeth=Zero  SaturateOnIntegerOverflow=on
  b(1)(1) : Gain  Gain=0.996982653533543983  ParamDataTypeStr=fixdt(1,16,15)  OutDataTypeStr=fixdt(1,32,30)  RndMeth=Zero  SaturateOnIntegerOverflow=on
  b(2)(1) : Gain  Gain=-0.996982653533543983  ParamDataTypeStr=fixdt(1,16,15)  OutDataTypeStr=fixdt(1,32,30)  RndMeth=Zero  SaturateOnIntegerOverflow=on
  s(2) : Gain  Gain=0.99999999999983169  ParamDataTypeStr=fixdt(1,16,15)  OutDataTypeStr=fixdt(1,16,11)  RndMeth=Zero  SaturateOnIntegerOverflow=on
  Output : Outport
  wires:
  Input/1 -> ConvertIn/1
  ConvertScale1/1 -> b(1)(1)/1, B2Delay1/1
  b(1)(1)/1 -> SumB21/1
  SumB21/1 -> SumA21/1
  SumA21/1 -> CastStates1/1
  CastStates1/1 -> s(2)/1, A2Delay1/1
  B2Delay1/1 -> b(2)(1)/1
  b(2)(1)/1 -> SumB21/2
  a(2)(1)/1 -> SumA21/2
  A2Delay1/1 -> a(2)(1)/1
  s(2)/1 -> Output/1
  ConvertIn/1 -> ConvertScale1/1

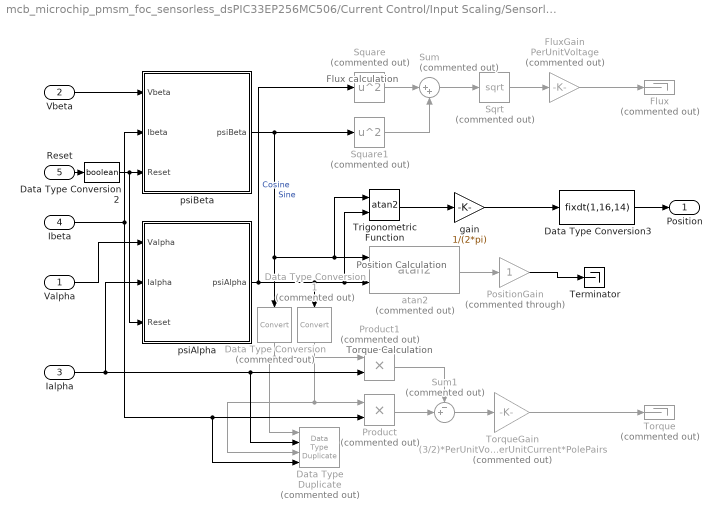
== system mcb_microchip_pmsm_foc_sensorless_dsPIC33EP256MC506/Current Control/Input Scaling/Sensorless/Flux Observer2 ==
  note: Flux calculation
  note: Position Calculation
  note: Torque Calculation
  Valpha : Inport  SampleTime=BlockSampleTime
  Vbeta : Inport  Port=2  SampleTime=BlockSampleTime
  Ialpha : Inport  Port=3  SampleTime=BlockSampleTime
  Ibeta : Inport  Port=4  SampleTime=BlockSampleTime
  Reset : Inport  Port=5  SampleTime=BlockSampleTime
  Data Type Duplicate : DataTypeDuplicate  Commented=on  NumInputPorts=4
  Data Type Conversion : DataTypeConversion  Commented=on  RndMeth=Simplest
  Data Type Conversion1 : DataTypeConversion  Commented=on  RndMeth=Simplest
  Data Type Conversion2 : DataTypeConversion  OutDataTypeStr=boolean  RndMeth=Simplest
  Data Type Conversion3 : DataTypeConversion  OutDataTypeStr=fixdt(1,16,14)  RndMeth=Simplest
  Flux : Terminator  Commented=on
  FluxGain : Gain  Commented=on  Gain=PerUnitVoltage  OutDataTypeStr=FluxDatatype  RndMeth=Simplest
  PositionGain : Gain  Commented=through  OutDataTypeStr=PositionDatatype  RndMeth=Simplest
  Product : Product  Commented=on  RndMeth=Simplest  OutDataTypeStr=Inherit: Same as first input
  Product1 : Product  Commented=on  RndMeth=Simplest  OutDataTypeStr=Inherit: Same as first input
  Sqrt : Sqrt  Commented=on  RndMeth=Simplest  IntermediateResultsDataTypeStr=Inherit: Inherit from input  SaturateOnIntegerOverflow=on
  Square : Math  Commented=on  Operator=square  RndMeth=Simplest  SaturateOnIntegerOverflow=on
  Square1 : Math  Commented=on  Operator=square  RndMeth=Simplest  SaturateOnIntegerOverflow=on
  Sum : Sum  Commented=on  Inputs=|++
  Sum1 : Sum  Commented=on  Inputs=-+|
  Terminator : Terminator
  Torque : Terminator  Commented=on
  TorqueGain : Gain  Commented=on  Gain=(3/2)*PerUnitVoltage*PerUnitCurrent*PolePairs  OutDataTypeStr=TorqueDatatype
  Trigonometric Function : Trigonometry  Operator=atan2  ApproximationMethod=CORDIC
  atan2 : mcbcontrolslib/atan2  Commented=on  outputUnit=PerUnit
      settings: SourceProductBaseCode=MT
  gain : Gain  Gain=1/(2*pi)  OutDataTypeStr=fixdt(0,16,16)  RndMeth=Simplest
  psiAlpha : Subsystem
  psiBeta : Subsystem
  Position : Outport
  wires:
  Data Type Conversion2/1 -> psiBeta/3(Reset), psiAlpha/3(Reset)
  Data Type Conversion1/1 -> Product/1, Data Type Duplicate/3
  Data Type Conversion/1 -> Product1/1, Data Type Duplicate/1
  atan2/1 -> PositionGain/1
  Sqrt/1 -> FluxGain/1
  Square1/1 -> Sum/2
  Sum/1 -> Sqrt/1
  Square/1 -> Sum/1
  FluxGain/1 -> Flux/1
  Sum1/1 -> TorqueGain/1
  Product1/1 -> Sum1/1
  Ialpha/1 -> Product1/2, Data Type Duplicate/2, psiAlpha/2(Ialpha)
  Product/1 -> Sum1/2
  TorqueGain/1 -> Torque/1
  Reset/1 -> Data Type Conversion2/1
  Vbeta/1 -> psiBeta/1(Vbeta)
  Ibeta/1 -> Product/2, Data Type Duplicate/4, psiBeta/2(Ibeta)
  Valpha/1 -> psiAlpha/1(Valpha)
  PositionGain/1 -> Terminator/1
  Trigonometric Function/1 -> gain/1
  gain/1 -> Data Type Conversion3/1
  Data Type Conversion3/1 -> Position/1
  psiBeta/1(psiBeta) -> Data Type Conversion/1, atan2/1, Trigonometric Function/1, Square1/1  "Sine"
  psiAlpha/1(psiAlpha) -> Square/1, Data Type Conversion1/1, Trigonometric Function/2, atan2/2  "Cosine"

== system mcb_microchip_pmsm_foc_sensorless_dsPIC33EP256MC506/Current Control/Input Scaling/Sensorless/Speed Measurement2 ==
  note: Speed measurement
  note: Speed measurement
  Position : Inport  SampleTime=SampleTimeAsync
  Data Type Conversion1 : DataTypeConversion  OutDataTypeStr=int32  ConvertRealWorld=Stored Integer (SI)
  Delay : Delay  Commented=on  DelayLength=DelayLength  UseCircularBuffer=on
  Delay1 : Delay  DelayLength=DelayLength  UseCircularBuffer=on
  Shift Arithmetic1 : ArithShift  BinPtShiftNumber=14  BitShiftDirection=Left
  Shift Arithmetic2 : ArithShift  BitShiftNumber=18  BitShiftDirection=Left
  SpeedCount : Sum  Commented=on  Inputs=+-|  OutDataTypeStr=int32  RndMeth=Simplest
  SpeedCount1 : Sum  Inputs=+-|  OutDataTypeStr=int32  RndMeth=Simplest
  SpeedGain : Gain  Commented=on  Gain=60/(DelayLength*SampleTimeAsync(1)*PU_System.N_base*4294967296)  ParamDataTypeStr=fixdt(0,16)  OutDataTypeStr=fixdt(1,16,12)  RndMeth=Simplest
  SpeedGain1 : Gain  Gain=60/(DelayLength*SampleTimeAsync(1)*PU_System.N_base*4294967296)  ParamDataTypeStr=fixdt(0,16)  OutDataTypeStr=fixdt(1,16,12)  RndMeth=Simplest
  SpeedToCount : Gain  Commented=on  Gain=uint32(4294967296/1)  ParamDataTypeStr=uint32  OutDataTypeStr=uint32  RndMeth=Simplest
  Speed : Outport  VectorParamsAs1DForOutWhenUnconnected=off
  wires:
  Data Type Conversion1/1 -> Shift Arithmetic2/1
  Shift Arithmetic1/1 -> Data Type Conversion1/1
  Position/1 -> SpeedToCount/1, Shift Arithmetic1/1
  Delay1/1 -> SpeedCount1/2
  Shift Arithmetic2/1 -> SpeedCount1/1, Delay1/1
  SpeedCount1/1 -> SpeedGain1/1
  SpeedCount/1 -> SpeedGain/1
  SpeedToCount/1 -> Delay/1, SpeedCount/1
  Delay/1 -> SpeedCount/2
  SpeedGain1/1 -> Speed/1

== system mcb_microchip_pmsm_foc_sensorless_dsPIC33EP256MC506/Current Control/Output Scaling/Mode Selector/Subsystem1 ==
  Count : Inport
  Compare To Constant : simulink/Logic and Bit Operations/Compare To Constant  relop=>=  const=1  OutDataTypeStr=boolean
  Compare To Constant1 : simulink/Logic and Bit Operations/Compare To Constant  relop=<  const=1  OutDataTypeStr=boolean
  Data Store Write1 : DataStoreWrite  DataStoreName=EnableFOC  IndexOptions=Index vector (dialog)  Indices=1  OutputSizes=1
  Gain : Gain  Gain=1/(2*PWM_frequency)  OutDataTypeStr=dataType2  RndMeth=Simplest
  Current Offset : Outport
  EnClosedLoop : Outport  Port=2
  tag scope: EnCurOffset=global
  wires:
  Count/1 -> Gain/1
  Gain/1 -> Compare To Constant1/1, Compare To Constant/1
  Compare To Constant/1 -> Data Store Write1/1, EnClosedLoop/1
  Compare To Constant1/1 -> [EnCurOffset], Current Offset/1

== system mcb_microchip_pmsm_foc_sensorless_dsPIC33EP256MC506/Current Control/Output Scaling/Mode Selector/Up Counter ==
  Enable : EnablePort  StatesWhenEnabling=reset
  Add1 : Sum  SaturateOnIntegerOverflow=on
  Constant : Constant  OutDataTypeStr=uint32
  Delay : Delay  DelayLength=1
  Count : Outport  InitialOutput=0
  wires:
  Delay/1 -> Add1/2
  Add1/1 -> Count/1, Delay/1
  Constant/1 -> Add1/1

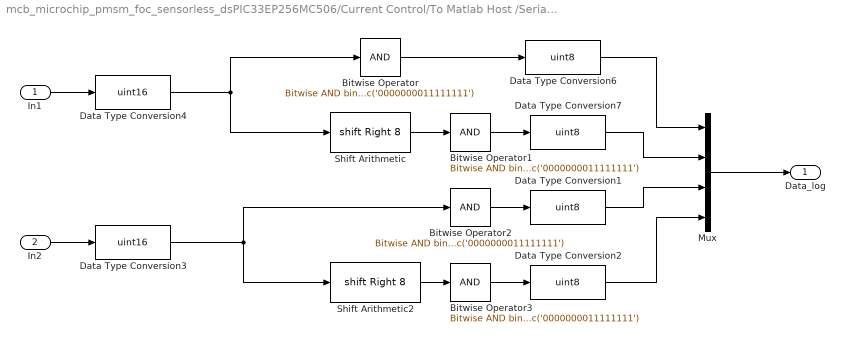
== system mcb_microchip_pmsm_foc_sensorless_dsPIC33EP256MC506/Current Control/To Matlab Host /Serial Send/Debug_Data ==
  In1 : Inport
  In2 : Inport  Port=2
  Bitwise Operator{,1..3} (4 alike) : simulink/Logic and Bit Operations/Bitwise Operator  logicop=AND  UseBitMask=on  BitMask=bin2dec('0000000011111111')  BitMaskRealWorld=Stored Integer
  Data Type Conversion{1..2,6..7} (4 alike) : DataTypeConversion  OutDataTypeStr=uint8  RndMeth=Simplest
  Data Type Conversion3 : DataTypeConversion  OutDataTypeStr=uint16  ConvertRealWorld=Stored Integer (SI)  RndMeth=Simplest
  Data Type Conversion4 : DataTypeConversion  OutDataTypeStr=uint16  ConvertRealWorld=Stored Integer (SI)  RndMeth=Simplest
  Mux : Mux
  Shift Arithmetic : ArithShift  BitShiftNumber=8  BitShiftDirection=Right
  Shift Arithmetic2 : ArithShift  BitShiftNumber=8  BitShiftDirection=Right
  Data_log : Outport
  wires:
  Data Type Conversion3/1 -> Bitwise Operator2/1, Shift Arithmetic2/1
  Bitwise Operator3/1 -> Data Type Conversion2/1
  Shift Arithmetic2/1 -> Bitwise Operator3/1
  Bitwise Operator1/1 -> Data Type Conversion7/1
  Data Type Conversion2/1 -> Mux/4
  Shift Arithmetic/1 -> Bitwise Operator1/1
  Bitwise Operator/1 -> Data Type Conversion6/1
  Data Type Conversion1/1 -> Mux/3
  Bitwise Operator2/1 -> Data Type Conversion1/1
  Data Type Conversion7/1 -> Mux/2
  Data Type Conversion6/1 -> Mux/1
  Data Type Conversion4/1 -> Shift Arithmetic/1, Bitwise Operator/1
  In1/1 -> Data Type Conversion4/1
  In2/1 -> Data Type Conversion3/1
  Mux/1 -> Data_log/1

== system mcb_microchip_pmsm_foc_sensorless_dsPIC33EP256MC506/Current Control/To Matlab Host /Serial Send/SCI_Tx ==
  note: Fast Serial Data Monitoring (32-bit)
  Data_Log : Inport
  Counter Limited : simulink/Sources/Counter Limited  uplimit=599  tsamp=-1
  Data : Subsystem  TreatAsAtomicUnit=on
  End : Subsystem  TreatAsAtomicUnit=on
  If : If  IfExpression=u1 == 0  ElseIfExpressions=u1 == 599
  Start : Subsystem  TreatAsAtomicUnit=on
  wires:
  If/3 -> Data/Action
  Counter Limited/1 -> If/1
  If/2 -> End/Action
  If/1 -> Start/Action
  Data_Log/1 -> End/1(Data), Start/1(Data), Data/1(Data)

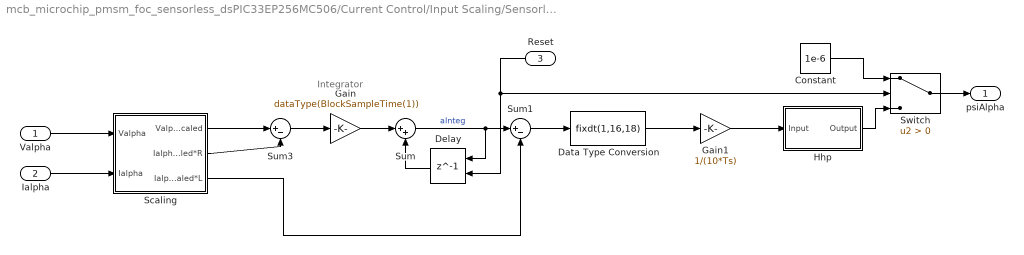
== system mcb_microchip_pmsm_foc_sensorless_dsPIC33EP256MC506/Current Control/Input Scaling/Sensorless/Flux Observer2/psiAlpha ==
  note: Integrator
  Valpha : Inport
  Ialpha : Inport  Port=2
  Reset : Inport  Port=3
  Constant : Constant  Value=1e-6  OutDataTypeStr=Inherit: Inherit via back propagation
  Data Type Conversion : DataTypeConversion  OutDataTypeStr=fixdt(1,16,18)  RndMeth=Zero
  Delay : Delay  DelayLength=1  ExternalReset=Level
      settings: InputPortMap=u0,r5
  Gain : Gain  Gain=dataType(BlockSampleTime(1))  ParamDataTypeStr=Inherit: Inherit from 'Gain'  OutDataTypeStr=fixdt(1,32,24)  RndMeth=Zero  SaturateOnIntegerOverflow=on
  Gain1 : Gain  Gain=1/(10*Ts)  OutDataTypeStr=fixdt(1,16,13)  RndMeth=Zero
  Hhp : Subsystem  Tag=FilterWizardSubSystem
  Scaling : Subsystem
  Sum : Sum  Inputs=|++  RndMeth=Zero  SaturateOnIntegerOverflow=on  OutDataTypeStr=Inherit: Same as first input
  Sum1 : Sum  Inputs=|+-  RndMeth=Zero  SaturateOnIntegerOverflow=on  OutDataTypeStr=Inherit: Same as first input
  Sum3 : Sum  Inputs=|+-  RndMeth=Zero  OutDataTypeStr=Inherit: Same as first input
  Switch : Switch  Criteria=u2 > Threshold
  psiAlpha : Outport
  wires:
  Switch/1 -> psiAlpha/1
  Constant/1 -> Switch/1
  Reset/1 -> Delay/2, Switch/2
  Scaling/3(IalphaScaled*L) -> Sum1/2
  Gain/1 -> Sum/1
  Sum3/1 -> Gain/1
  Delay/1 -> Sum/2
  Scaling/2(IalphaScaled*R) -> Sum3/2
  Scaling/1(ValphaScaled) -> Sum3/1
  Ialpha/1 -> Scaling/2(Ialpha)
  Valpha/1 -> Scaling/1("Valpha ")
  Gain1/1 -> Hhp/1(Input)
  Sum1/1 -> Data Type Conversion/1
  Data Type Conversion/1 -> Gain1/1
  Hhp/1(Output) -> Switch/3
  Sum/1 -> Delay/1, Sum1/1  "aInteg"
